simulink model "sxxxxxx_sim"  (R2025b)
settings: Solver=VariableStepAuto  StartTime=0.0  StopTime=t_sim  RelTol=1e-3
values from neighbouring files (symbols this model uses):
  delta_2 = 1    [sxxxxxx_Design.m]
  rho = 0    [sxxxxxx_Design.m]
  Ts = 10e-3    (= 0.01)    [sxxxxxx_Design.m]
libraries: cstblocks x2, simulink x1
settings Model: Creator=davidecovolo  LastModifiedBy=davidecovolo

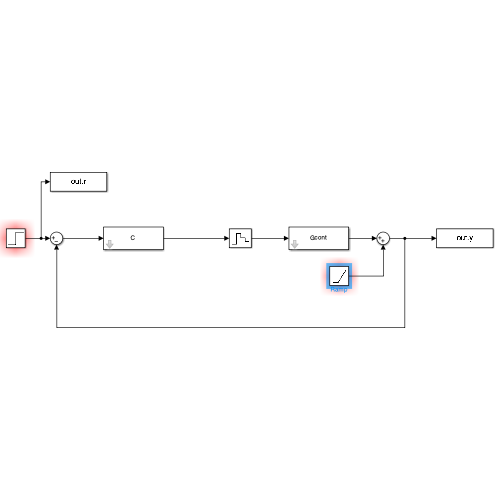
[thumbnail: Simulink's stored preview of the top-level diagram]
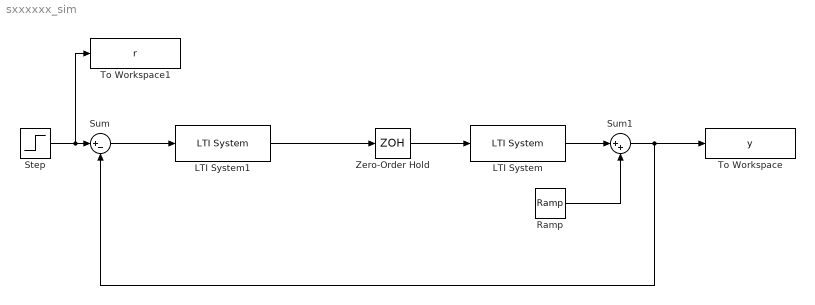
== system sxxxxxx_sim ==
  LTI System : cstblocks/LTI System  sys=Gcont  IC=[]  PadeOrder=0
  LTI System1 : cstblocks/LTI System  sys=C  IC=[]  PadeOrder=0
  Ramp : simulink/Sources/Ramp  slope=delta_2  start=0  InitialOutput=0
  Step : Step  Time=0  After=rho  SampleTime=0
  Sum : Sum  Inputs=|+-
  Sum1 : Sum  Inputs=|++
  To Workspace : ToWorkspace  VariableName=y  SaveFormat=Timeseries  SampleTime=-1
  To Workspace1 : ToWorkspace  VariableName=r  SaveFormat=Timeseries  SampleTime=-1
  Zero-Order Hold : ZeroOrderHold  SampleTime=Ts
  wires:
  Zero-Order Hold/1 -> LTI System/1
  LTI System1/1 -> Zero-Order Hold/1
  Sum/1 -> LTI System1/1
  Step/1 -> To Workspace1/1, Sum/1
  LTI System/1 -> Sum1/1
  Ramp/1 -> Sum1/2
  Sum1/1 -> To Workspace/1, Sum/2
